simulink model "SistemaA"  (R2019a)
settings: Solver=ode23t  StartTime=0.0  StopTime=10.0  MaxStep=1E-3  RelTol=1e-3
libraries: simulink x1
settings Model: LastModifiedBy=josu5
settings DataIOCC: ReturnWorkspaceOutputs=off  TimeSaveName=t
settings DebuggingCC: AlgebraicLoopMsg=none  ArtificialAlgebraicLoopMsg=none  MaxConsecutiveZCsMsg=none  UnconnectedInputMsg=none  UnconnectedOutputMsg=none  UnconnectedLineMsg=none
settings ModelReferenceCC: EnableRefExpFcnMdlSchedulingChecks=off
settings RTWCC: Description=Generic Real-Time Target

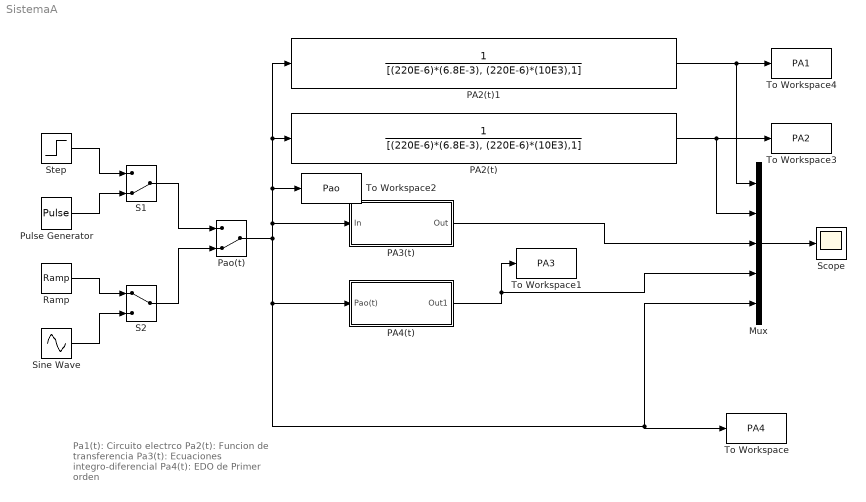
== system SistemaA ==
  note: Pa1(t): Circuito electrco
      | Pa2(t): Funcion de transferencia
      | Pa3(t): Ecuaciones integro-diferencial
      | Pa4(t): EDO de Primer orden
  Mux : Mux  Inputs=5
  PA2(t) : TransferFcn  Denominator=[(220E-6)*(6.8E-3), (220E-6)*(10E3),1]
  PA2(t)1 : TransferFcn  Denominator=[(220E-6)*(6.8E-3), (220E-6)*(10E3),1]
  PA3(t) : Subsystem
  PA4(t) : Subsystem
  Pao(t) : ManualSwitch  CurrentSetting=0
  Pulse Generator : DiscretePulseGenerator  PulseType=Time based  Period=10  PulseWidth=10  PhaseDelay=1
  Ramp : simulink/Sources/Ramp  slope=1/10  start=0  InitialOutput=0
  S1 : ManualSwitch  CurrentSetting=0
  S2 : ManualSwitch
  Scope : Scope
  Sine Wave : Sin  Frequency=1.570  SampleTime=0.001
  Step : Step  Time=0  After=0.001  SampleTime=0
  To Workspace : ToWorkspace  VariableName=PA4  SaveFormat=Timeseries  SampleTime=-1
  To Workspace1 : ToWorkspace  VariableName=PA3  SaveFormat=Timeseries  SampleTime=-1
  To Workspace2 : ToWorkspace  VariableName=Pao  SaveFormat=Timeseries  SampleTime=-1
  To Workspace3 : ToWorkspace  VariableName=PA2  SaveFormat=Timeseries  SampleTime=-1
  To Workspace4 : ToWorkspace  VariableName=PA1  SaveFormat=Timeseries  SampleTime=-1
  wires:
  Ramp/1 -> S2/1
  Sine Wave/1 -> S2/2
  Step/1 -> S1/1
  Pulse Generator/1 -> S1/2
  S2/1 -> Pao(t)/2
  S1/1 -> Pao(t)/1
  Pao(t)/1 -> PA3(t)/1(In), To Workspace2/1, PA2(t)1/1, PA2(t)/1, PA4(t)/1(Pao(t)), To Workspace/1, Mux/5
  PA4(t)/1(Out1) -> To Workspace1/1, Mux/4
  Mux/1 -> Scope/1
  PA3(t)/1(Out) -> Mux/3
  PA2(t)/1 -> To Workspace3/1, Mux/2
  PA2(t)1/1 -> To Workspace4/1, Mux/1

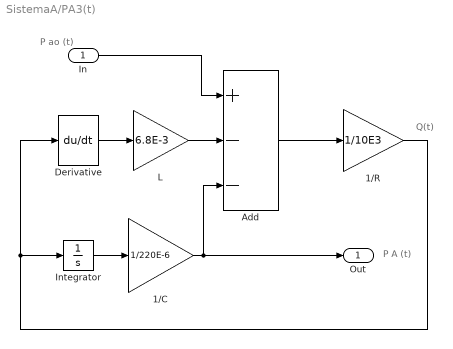
== system SistemaA/PA3(t) ==
  note: P ao (t)
  note: P A (t)
  note: Q(t)
  In : Inport
  1/C : Gain  Gain=1/220E-6
  1/R : Gain  Gain=1/10E3
  Add : Sum  Inputs=+--
  Derivative : Derivative
  Integrator : Integrator
  L : Gain  Gain=6.8E-3
  Out : Outport  VectorParamsAs1DForOutWhenUnconnected=on
  wires:
  Add/1 -> 1/R/1
  In/1 -> Add/1
  Integrator/1 -> 1/C/1
  L/1 -> Add/2
  1/C/1 -> Out/1, Add/3
  Derivative/1 -> L/1
  1/R/1 -> Derivative/1, Integrator/1

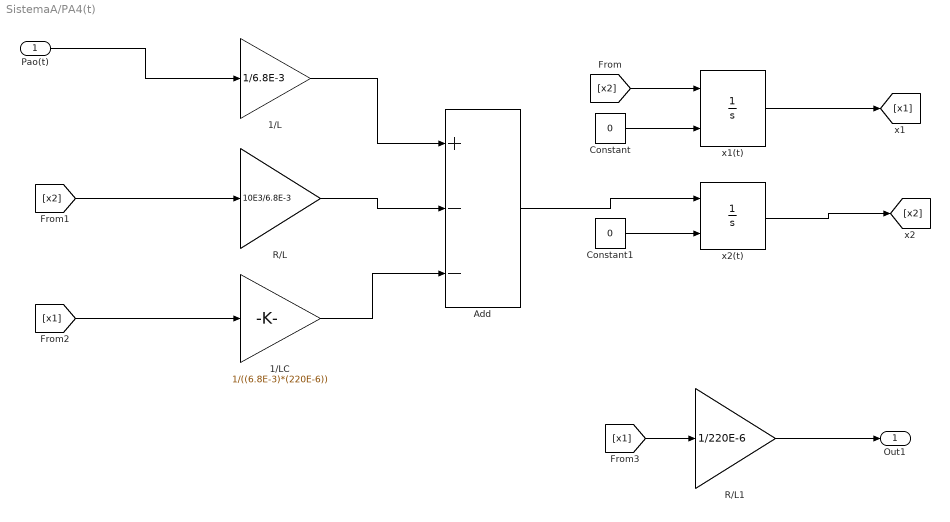
== system SistemaA/PA4(t) ==
  Pao(t) : Inport
  1/L : Gain  Gain=1/6.8E-3
  1/LC : Gain  Gain=1/((6.8E-3)*(220E-6))
  Add : Sum  Inputs=+--
  Constant : Constant  Value=0
  Constant1 : Constant  Value=0
  R/L : Gain  Gain=10E3/6.8E-3
  R/L1 : Gain  Gain=1/220E-6
  x1(t) : Integrator  InitialConditionSource=external
  x2(t) : Integrator  InitialConditionSource=external
  Out1 : Outport  VectorParamsAs1DForOutWhenUnconnected=on
  wires:
  x1(t)/1 -> [x1]
  [x2] -> x1(t)/1
  Constant/1 -> x1(t)/2
  Constant1/1 -> x2(t)/2
  1/L/1 -> Add/1
  R/L/1 -> Add/2
  1/LC/1 -> Add/3
  Add/1 -> x2(t)/1
  x2(t)/1 -> [x2]
  Pao(t)/1 -> 1/L/1
  [x2] -> R/L/1
  [x1] -> 1/LC/1
  [x1] -> R/L1/1
  R/L1/1 -> Out1/1
